simulink model "S_Func"  (R2020a)
settings: Solver=VariableStepAuto  StartTime=0.0  StopTime=100  RelTol=1e-6
undefined symbols (not defined in the file or in its folder): a1, a2, g, k, m
settings Model: Creator=faith  LastModifiedBy=faith

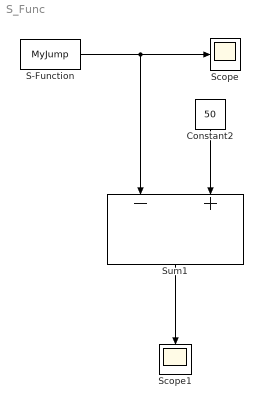
== system S_Func ==
  Constant2 : Constant  Value=50
  S-Function : S-Function  FunctionName=MyJump  Parameters=m,g,a1,a2,k  SFunctionDeploymentMode=off  EnableBusSupport=off
  Scope : Scope
  Scope1 : Scope
  Sum1 : Sum  Inputs=-+
  wires:
  Constant2/1 -> Sum1/2
  Sum1/1 -> Scope1/1
  S-Function/1 -> Sum1/1, Scope/1
